simulink model "simula_trajetoria_axebot_nao_linear_MPC_Otimo"  (Simulink 8.5)
settings: Solver=ode45  StartTime=0.0  StopTime=18  FixedStep=0.05  MaxStep=0.01  MinStep=1e-4  RelTol=1e-6
values from neighbouring files (symbols this model uses):
  Ac = diag([(Ae-Bv)/M (Ae-Bvn)/M (Ae*b*b - Bw)/J])    [robo_MPC.m]
  Ag = [Ad Z ; Cd*Ad I]    [robo_MPC.m]
  Bc = [0 sqrt(3)/(2*M) -sqrt(3)/(2*M) ; -1/M 1/(2*M) 1/(2*M) ; b/J b/J b/J]*Be    [robo_MPC.m]
  Bg = [Bd ; Cd*Bd]    [robo_MPC.m]
  deltaS = [deltaSv;deltaSvn;deltaSw]    [robo_MPC.m]
  Gc = Z    [robo_MPC.m]
  Kc = Z    [robo_MPC.m]
  N = 4    [robo_MPC.m]
  np = 0.0001    [robo_MPC.m]    (also in spline3d.m = 5)
  Thetaini = TrajTheta(1)    [init.m]    (also in spline3d.m)
  TrajPoints = 68    [init.m]    (also in spline3d.m = size(TrajX(:,1),1))
  TrajTheta = [TrajTheta atan2((0.5*sin(deg)+ 1.0),(0.5*cos(deg)+ 2.1)) ]    [init.m]    (also in spline3d.m = steta')
  TrajX = [TrajX (0.5*cos(deg)+ 2.1)]*4    [init.m]    (also in spline3d.m = sx')
  TrajY = [TrajY (0.5*sin(deg)+ 1.0)]*4    [init.m]    (also in spline3d.m = sy')
  ts = 0.05    [robo_MPC.m]
  Vnav = 0.3    [robo_MPC.m]
  Vs = [Vsv;Vsvn;Vsw]    [robo_MPC.m]
  Xini = TrajX(1)    [init.m]    (also in spline3d.m)
  Yini = TrajY(1)    [init.m]    (also in spline3d.m)
undefined symbols (not defined in the file or in its folder): Cd
libraries: simulink x1, aerolibobsolete x1
settings Model: Creator=tito  LastModifiedBy=jessivaldo
settings DebuggingCC: SolverPrmCheckMsg=warning  FcnCallInpInsideContextMsg=UseLocalSettings

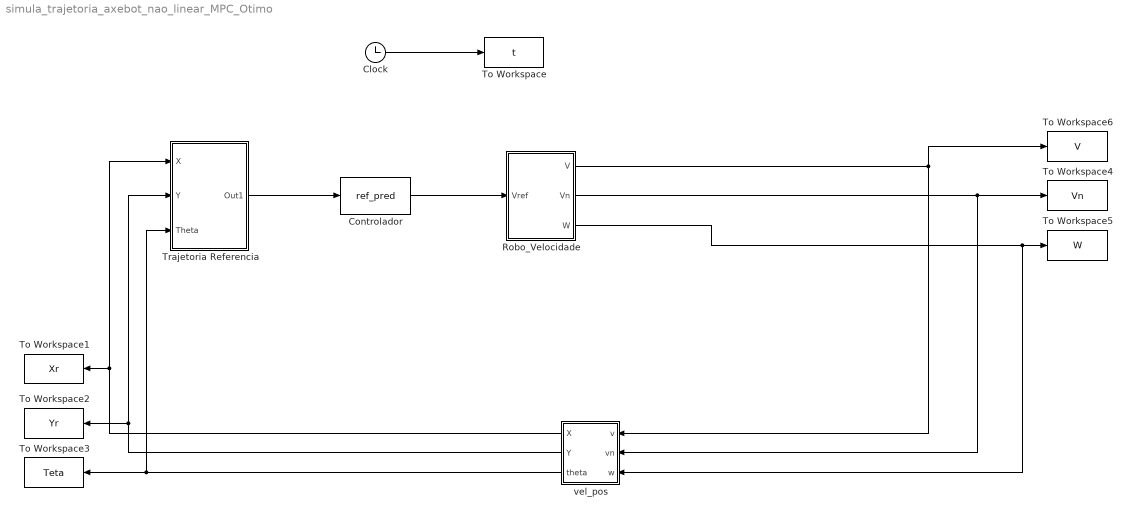
== system simula_trajetoria_axebot_nao_linear_MPC_Otimo ==
  Clock : Clock
  Controlador : S-Function  FunctionName=ref_pred  Parameters=TrajX,TrajY,TrajTheta,TrajPoints
  Robo_Velocidade : Subsystem
  To Workspace : ToWorkspace  VariableName=t  SampleTime=ts
  To Workspace1 : ToWorkspace  VariableName=Xr  SampleTime=ts
  To Workspace2 : ToWorkspace  VariableName=Yr  SampleTime=ts
  To Workspace3 : ToWorkspace  VariableName=Teta  SampleTime=ts
  To Workspace4 : ToWorkspace  VariableName=Vn  SampleTime=ts
  To Workspace5 : ToWorkspace  VariableName=W  SampleTime=ts
  To Workspace6 : ToWorkspace  VariableName=V  SampleTime=ts
  Trajetoria Referencia : Subsystem
  vel_pos : Subsystem
  wires:
  Clock/1 -> To Workspace/1
  Robo_Velocidade/1(V) -> To Workspace6/1, vel_pos/1(v)
  Robo_Velocidade/2(Vn) -> vel_pos/2(vn), To Workspace4/1
  Trajetoria Referencia/1(Out1) -> Controlador/1
  vel_pos/1(X) -> To Workspace1/1, Trajetoria Referencia/1(X)
  vel_pos/2(Y) -> To Workspace2/1, Trajetoria Referencia/2(Y)
  Robo_Velocidade/3(W) -> vel_pos/3(w), To Workspace5/1
  Controlador/1 -> Robo_Velocidade/1(Vref)
  vel_pos/3(theta) -> To Workspace3/1, Trajetoria Referencia/3(Theta)

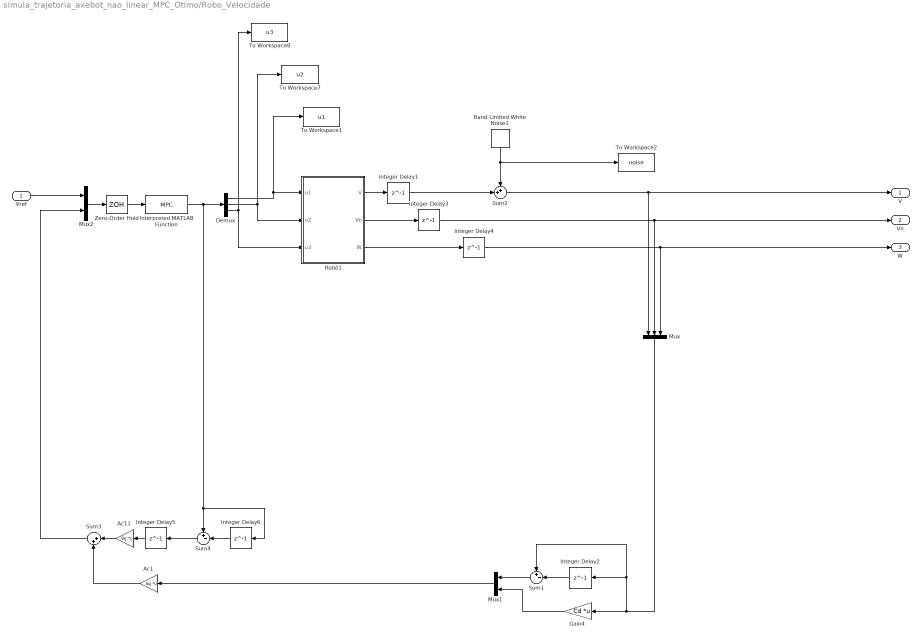
== system simula_trajetoria_axebot_nao_linear_MPC_Otimo/Robo_Velocidade ==
  Vref : Inport
  Ac1 : Gain  Gain=Ag  Multiplication=Matrix(K*u)
  Ac11 : Gain  Gain=Bg  Multiplication=Matrix(K*u)
  Band-Limited White Noise1 : simulink/Sources/Band-Limited White Noise  Cov=[np]  Ts=ts  seed=[23341]
  Demux : Demux  Outputs=3
  Gain4 : Gain  Gain=Cd  Multiplication=Matrix(K*u)  SampleTime=ts
  Integer Delay{1..6} (6 alike) : Delay  DelayLength=1  InputProcessing=Inherited  SampleTime=ts
  Interpreted MATLAB Function : MATLABFcn  MATLABFcn=MPC  OutputDimensions=3
  Mux : Mux  Inputs=3
  Mux1 : Mux  Inputs=2
  Mux2 : Mux  Inputs=2
  Robô1 : Subsystem
  Sum1 : Sum  Inputs=+-|
  Sum2 : Sum  Inputs=++|
  Sum3 : Sum  Inputs=|++
  Sum4 : Sum  Inputs=+-|
  To Workspace1 : ToWorkspace  VariableName=u1  SampleTime=ts
  To Workspace2 : ToWorkspace  VariableName=noise  SampleTime=ts
  To Workspace7 : ToWorkspace  VariableName=u2  SampleTime=ts
  To Workspace8 : ToWorkspace  VariableName=u3  SampleTime=ts
  Zero-Order Hold : ZeroOrderHold  SampleTime=ts
  V : Outport
  Vn : Outport  Port=2
  W : Outport  Port=3
  wires:
  Sum1/1 -> Mux1/1
  Gain4/1 -> Mux1/2
  Integer Delay2/1 -> Sum1/2
  Band-Limited White Noise1/1 -> Sum2/1, To Workspace2/1
  Vref/1 -> Mux2/1
  Demux/2 -> To Workspace7/1, Robô1/2(u2)
  Demux/3 -> To Workspace8/1, Robô1/3(u3)
  Robô1/1(V) -> Integer Delay1/1
  Mux/1 -> Sum1/1, Integer Delay2/1, Gain4/1
  Demux/1 -> Robô1/1(u1), To Workspace1/1
  Robô1/2(Vn) -> Integer Delay3/1
  Integer Delay3/1 -> Vn/1, Mux/2
  Robô1/3(W) -> Integer Delay4/1
  Integer Delay4/1 -> W/1, Mux/3
  Mux2/1 -> Zero-Order Hold/1
  Zero-Order Hold/1 -> Interpreted MATLAB Function/1
  Integer Delay1/1 -> Sum2/2
  Sum2/1 -> Mux/1, V/1
  Mux1/1 -> Ac1/1
  Ac11/1 -> Sum3/1
  Integer Delay5/1 -> Ac11/1
  Sum4/1 -> Integer Delay5/1
  Ac1/1 -> Sum3/2
  Sum3/1 -> Mux2/2
  Integer Delay6/1 -> Sum4/2
  Interpreted MATLAB Function/1 -> Demux/1, Integer Delay6/1, Sum4/1

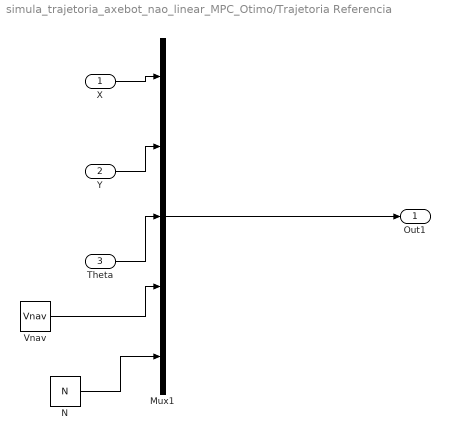
== system simula_trajetoria_axebot_nao_linear_MPC_Otimo/Trajetoria Referencia ==
  X : Inport
  Y : Inport  Port=2
  Theta : Inport  Port=3
  Mux1 : Mux  Inputs=5
  N : Constant  Value=N
  Vnav : Constant  Value=Vnav
  Out1 : Outport
  wires:
  Vnav/1 -> Mux1/4
  X/1 -> Mux1/1
  Y/1 -> Mux1/2
  Theta/1 -> Mux1/3
  Mux1/1 -> Out1/1
  N/1 -> Mux1/5

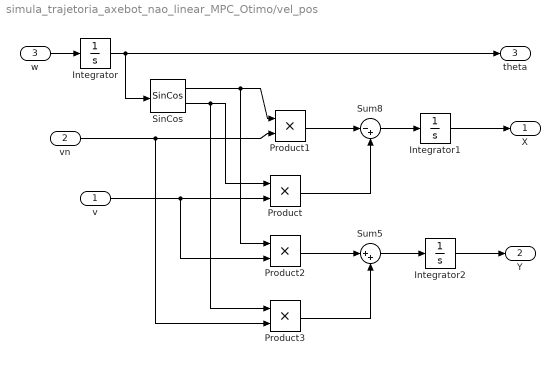
== system simula_trajetoria_axebot_nao_linear_MPC_Otimo/vel_pos ==
  v : Inport
  vn : Inport  Port=2
  w : Inport  Port=3
  Integrator : Integrator  InitialCondition=Thetaini
  Integrator1 : Integrator  InitialCondition=Xini
  Integrator2 : Integrator  InitialCondition=Yini
  Product{,1..3} (4 alike) : Product  RndMeth=Zero
  SinCos : aerolibobsolete/SinCos
  Sum5 : Sum  Inputs=|++
  Sum8 : Sum  Inputs=|-+
  X : Outport
  Y : Outport  Port=2
  theta : Outport  Port=3
  wires:
  Sum8/1 -> Integrator1/1
  Sum5/1 -> Integrator2/1
  Product3/1 -> Sum5/2
  Product2/1 -> Sum5/1
  Product1/1 -> Sum8/1
  Product/1 -> Sum8/2
  SinCos/1 -> Product2/1, Product1/1
  SinCos/2 -> Product3/1, Product/1
  Integrator/1 -> SinCos/1, theta/1
  Integrator1/1 -> X/1
  Integrator2/1 -> Y/1
  w/1 -> Integrator/1
  vn/1 -> Product1/2, Product3/2
  v/1 -> Product/2, Product2/2

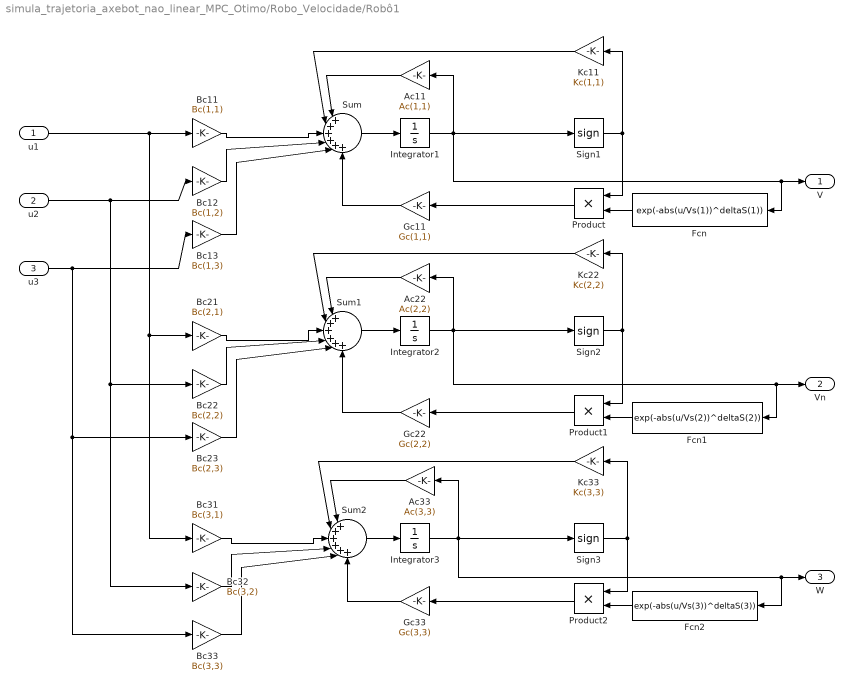
== system simula_trajetoria_axebot_nao_linear_MPC_Otimo/Robo_Velocidade/Robô1 ==
  u1 : Inport
  u2 : Inport  Port=2
  u3 : Inport  Port=3
  Ac11 : Gain  Gain=Ac(1,1)
  Ac22 : Gain  Gain=Ac(2,2)
  Ac33 : Gain  Gain=Ac(3,3)
  Bc11 : Gain  Gain=Bc(1,1)
  Bc12 : Gain  Gain=Bc(1,2)
  Bc13 : Gain  Gain=Bc(1,3)
  Bc21 : Gain  Gain=Bc(2,1)
  Bc22 : Gain  Gain=Bc(2,2)
  Bc23 : Gain  Gain=Bc(2,3)
  Bc31 : Gain  Gain=Bc(3,1)
  Bc32 : Gain  Gain=Bc(3,2)
  Bc33 : Gain  Gain=Bc(3,3)
  Fcn : Fcn  Expr=exp(-abs(u/Vs(1))^deltaS(1))
  Fcn1 : Fcn  Expr=exp(-abs(u/Vs(2))^deltaS(2))
  Fcn2 : Fcn  Expr=exp(-abs(u/Vs(3))^deltaS(3))
  Gc11 : Gain  Gain=Gc(1,1)
  Gc22 : Gain  Gain=Gc(2,2)
  Gc33 : Gain  Gain=Gc(3,3)
  Integrator1 : Integrator
  Integrator2 : Integrator
  Integrator3 : Integrator
  Kc11 : Gain  Gain=Kc(1,1)
  Kc22 : Gain  Gain=Kc(2,2)
  Kc33 : Gain  Gain=Kc(3,3)
  Product : Product  RndMeth=Zero
  Product1 : Product  RndMeth=Zero
  Product2 : Product  RndMeth=Zero
  Sign1 : Signum  ZeroCross=off
  Sign2 : Signum  ZeroCross=off
  Sign3 : Signum  ZeroCross=off
  Sum : Sum  Inputs=|++++++
  Sum1 : Sum  Inputs=|++++++
  Sum2 : Sum  Inputs=|++++++
  V : Outport
  Vn : Outport  Port=2
  W : Outport  Port=3
  wires:
  Gc33/1 -> Sum2/6
  Gc22/1 -> Sum1/6
  Gc11/1 -> Sum/6
  Fcn2/1 -> Product2/2
  Fcn1/1 -> Product1/2
  Fcn/1 -> Product/2
  Kc33/1 -> Sum2/2
  Kc22/1 -> Sum1/2
  Kc11/1 -> Sum/2
  Product2/1 -> Gc33/1
  Product1/1 -> Gc22/1
  Product/1 -> Gc11/1
  Bc33/1 -> Sum2/5
  Bc32/1 -> Sum2/4
  Bc31/1 -> Sum2/3
  Sign3/1 -> Product2/1, Kc33/1
  Ac33/1 -> Sum2/1
  Integrator3/1 -> Fcn2/1, W/1, Sign3/1, Ac33/1
  Sum2/1 -> Integrator3/1
  Bc23/1 -> Sum1/5
  Bc22/1 -> Sum1/4
  Bc21/1 -> Sum1/3
  Sign2/1 -> Product1/1, Kc22/1
  Ac22/1 -> Sum1/1
  Integrator2/1 -> Fcn1/1, Vn/1, Sign2/1, Ac22/1
  Sum1/1 -> Integrator2/1
  Bc13/1 -> Sum/5
  Bc12/1 -> Sum/4
  Bc11/1 -> Sum/3
  Sign1/1 -> Product/1, Kc11/1
  Ac11/1 -> Sum/1
  Integrator1/1 -> Fcn/1, V/1, Sign1/1, Ac11/1
  Sum/1 -> Integrator1/1
  u3/1 -> Bc33/1, Bc23/1, Bc13/1
  u2/1 -> Bc32/1, Bc22/1, Bc12/1
  u1/1 -> Bc31/1, Bc21/1, Bc11/1
